simulink model "two_sub_model"  (Simulink 8.4)
settings: Solver=FixedStepDiscrete  StartTime=0.0  StopTime="                                                                                 300"  FixedStep=1/256  RelTol=1e-3
undefined symbols (not defined in the file): currentCFG_one_sub_model_UB, UB
libraries: gRTanalyze x6, gUSBamplib x2, Tools x1
settings Model: Creator=2110973l  LastModifiedBy=2110973l
settings DataIOCC: SignalLoggingSaveFormat=Dataset
settings OptimizationCC: ExpressionDepthLimit=128
settings DebuggingCC: UnderspecifiedInitializationDetection=Simplified  MergeDetectMultiDrivingBlocksExec=error  FcnCallInpInsideContextMsg=EnableAllAsError  StateNameClashWarn=none
settings GRTTargetCC: CombineOutputUpdateFcns=on  GRTInterface=off

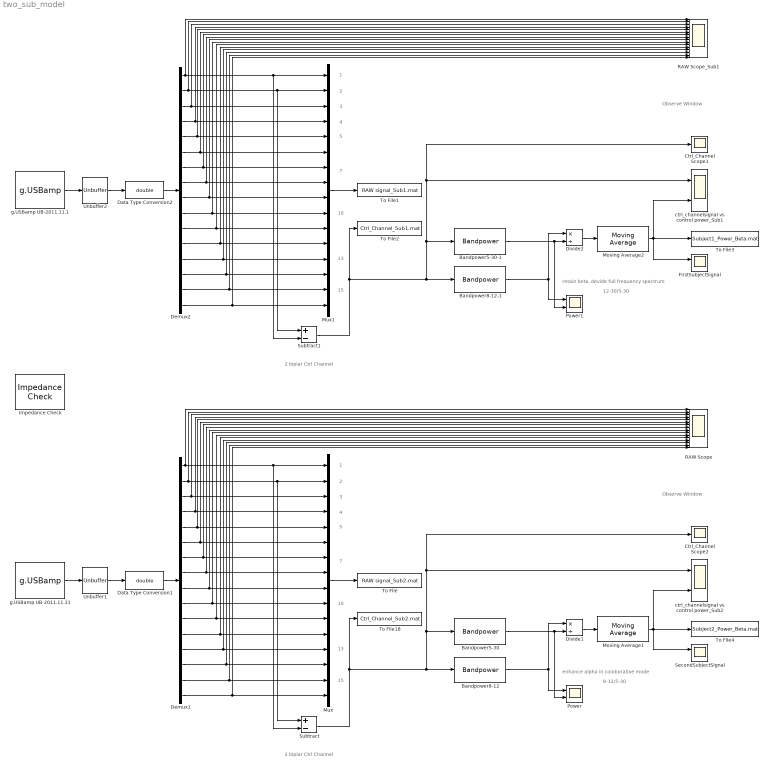
== system two_sub_model ==
  note: 13
  note: 15
  note: 4
  note: 3
  note: 7
  note: 10
  note: 5
  note: 2
  note: 1
  note: Observe Window
  note: 2 biplar Ctrl Channel
  note: enhance alpha in coloborative mode
  note: 8-12/5-30
  note: 13
  note: 15
  note: 4
  note: 3
  note: 7
  note: 10
  note: 5
  note: 2
  note: 1
  note: Observe Window
  note: 2 biplar Ctrl Channel
  note: retain beta, devide full frequency spectrum
  note: 12-30/5-30
  Bandpower5-30 : gRTanalyze/Bandpower  Order=5  LowerFreq=5  UpperFreq=30  WindowLength=128
  Bandpower5-30-1 : gRTanalyze/Bandpower  Order=5  LowerFreq=5  UpperFreq=30  WindowLength=128
  Bandpower8-12 : gRTanalyze/Bandpower  Order=5  LowerFreq=8  UpperFreq=12  WindowLength=128
  Bandpower8-12-1 : gRTanalyze/Bandpower  Order=5  LowerFreq=8  UpperFreq=12  WindowLength=128
  Ctrl_Channel Scope1 : Scope
      settings: YMin=-100  YMax=100  SaveName=ScopeData2
  Ctrl_Channel Scope2 : Scope
      settings: YMin=-100  YMax=100
  Data Type Conversion1 : DataTypeConversion  OutDataTypeStr=double
  Data Type Conversion2 : DataTypeConversion  OutDataTypeStr=double
  Demux1 : Demux  Outputs=16
  Demux2 : Demux  Outputs=16
  Divide1 : Product  Inputs=*/
  Divide2 : Product  Inputs=*/
  FirstSubjectSignal : Scope  NumInputPorts=2
      settings: YMin=1.014~-1  YMax=1.032~1  SaveName=ScopeData8
  Impedance Check : Tools/Impedance Check  SystemSampleTime=-1
  Moving Average1 : gRTanalyze/Moving Average  windowSize=256
  Moving Average2 : gRTanalyze/Moving Average  windowSize=256
  Mux : Mux  Inputs=16
  Mux1 : Mux  Inputs=16
  Power : Scope  NumInputPorts=2
      settings: YMin=0~0  YMax=1200~1200  SaveName=ScopeData5
  Power1 : Scope  NumInputPorts=2
      settings: YMin=0~0  YMax=1200~1200  SaveName=ScopeData4
  RAW Scope : Scope  NumInputPorts=16
      settings: YMin=-50~-50~-50~-50~-50~-50~-50~-50~-50~-50~-50~-50~-100~-50~-100~-100  YMax=50~50~50~50~50~50~50~50~50~50~50~50~100~50~100~100
  RAW Scope_Sub1 : Scope  NumInputPorts=16
      settings: YMin=-50~-50~-50~-50~-50~-50~-50~-50~-50~-50~-50~-50~-100~-50~-100~-100  YMax=50~50~50~50~50~50~50~50~50~50~50~50~100~50~100~100  SaveName=ScopeData6
  SecondSubjectSignal : Scope  NumInputPorts=2
      settings: YMin=1.014~-1  YMax=1.032~1  SaveName=ScopeData3
  Subtract : Sum  Inputs=+-
  Subtract1 : Sum  Inputs=+-
  To File : ToFile  Filename=RAW signal_Sub2.mat  MatrixName=AllChannel
  To File1 : ToFile  Filename=RAW signal_Sub1.mat  MatrixName=AllChannel
  To File18 : ToFile  Filename=Ctrl_Channel_Sub2.mat  MatrixName=Ctrl_Channel
  To File2 : ToFile  Filename=Ctrl_Channel_Sub1.mat  MatrixName=Ctrl_Channel
  To File3 : ToFile  Filename=Subject1_Power_Beta.mat  MatrixName=Subject1_Power_Beta
  To File4 : ToFile  Filename=Subject2_Power_Beta.mat  MatrixName=Subject2_Power_Beta
  Unbuffer1 : Unbuffer  SampleBasedProcessing=Same as frame based
  Unbuffer2 : Unbuffer  SampleBasedProcessing=Same as frame based
  ctrl_channelsignal vs control power_Sub1 : Scope  NumInputPorts=2
      settings: YMin=-100~0  YMax=100~20  SaveName=ScopeData9
  ctrl_channelsignal vs control power_Sub2 : Scope  NumInputPorts=2
      settings: YMin=-100~0  YMax=100~20  SaveName=ScopeData7
  g.USBamp UB-2011.11.1 : gUSBamplib/g.USBamp  cfg=currentCFG_one_sub_model_UB-2011.11.31.cfg  snr=UB-2011.11.31
  g.USBamp UB-2011.11.31 : gUSBamplib/g.USBamp  cfg=currentCFG_one_sub_model_UB-2011.11.31.cfg  snr=UB-2011.11.31
  wires:
  Bandpower8-12/1 -> Divide1/1, Power/1
  Bandpower5-30/1 -> Divide1/2, Power/2
  Moving Average1/1 -> To File4/1, ctrl_channelsignal vs control power_Sub2/2, SecondSubjectSignal/1
  Divide1/1 -> Moving Average1/1
  g.USBamp UB-2011.11.31/1 -> Unbuffer1/1
  Unbuffer1/1 -> Data Type Conversion1/1
  Data Type Conversion1/1 -> Demux1/1
  Demux1/11 -> RAW Scope/11, Mux/11
  Demux1/13 -> RAW Scope/13, Mux/13
  Demux1/15 -> RAW Scope/15, Mux/15
  Demux1/1 -> Subtract/2, Mux/1, RAW Scope/1
  Demux1/7 -> RAW Scope/7, Mux/7
  Demux1/9 -> RAW Scope/9, Mux/9
  Subtract/1 -> Bandpower8-12/1, Bandpower5-30/1, Ctrl_Channel Scope2/1, ctrl_channelsignal vs control power_Sub2/1, To File18/1
  Demux1/2 -> Subtract/1, Mux/2, RAW Scope/2
  Demux1/4 -> Mux/4, RAW Scope/4
  Demux1/6 -> RAW Scope/6, Mux/6
  Demux1/8 -> RAW Scope/8, Mux/8
  Demux1/12 -> RAW Scope/12, Mux/12
  Demux1/14 -> RAW Scope/14, Mux/14
  Demux1/16 -> RAW Scope/16, Mux/16
  Demux1/5 -> RAW Scope/5, Mux/5
  Demux1/3 -> Mux/3, RAW Scope/3
  Demux1/10 -> RAW Scope/10, Mux/10
  Mux/1 -> To File/1
  Bandpower8-12-1/1 -> Divide2/1, Power1/1
  Bandpower5-30-1/1 -> Divide2/2, Power1/2
  Moving Average2/1 -> To File3/1, ctrl_channelsignal vs control power_Sub1/2, FirstSubjectSignal/1
  Divide2/1 -> Moving Average2/1
  g.USBamp UB-2011.11.1/1 -> Unbuffer2/1
  Unbuffer2/1 -> Data Type Conversion2/1
  Data Type Conversion2/1 -> Demux2/1
  Demux2/11 -> RAW Scope_Sub1/11, Mux1/11
  Demux2/13 -> RAW Scope_Sub1/13, Mux1/13
  Demux2/15 -> RAW Scope_Sub1/15, Mux1/15
  Demux2/1 -> Subtract1/2, Mux1/1, RAW Scope_Sub1/1
  Demux2/7 -> RAW Scope_Sub1/7, Mux1/7
  Demux2/9 -> RAW Scope_Sub1/9, Mux1/9
  Subtract1/1 -> Bandpower8-12-1/1, Bandpower5-30-1/1, Ctrl_Channel Scope1/1, ctrl_channelsignal vs control power_Sub1/1, To File2/1
  Demux2/2 -> Subtract1/1, Mux1/2, RAW Scope_Sub1/2
  Demux2/4 -> Mux1/4, RAW Scope_Sub1/4
  Demux2/6 -> RAW Scope_Sub1/6, Mux1/6
  Demux2/8 -> RAW Scope_Sub1/8, Mux1/8
  Demux2/12 -> RAW Scope_Sub1/12, Mux1/12
  Demux2/14 -> RAW Scope_Sub1/14, Mux1/14
  Demux2/16 -> RAW Scope_Sub1/16, Mux1/16
  Demux2/5 -> RAW Scope_Sub1/5, Mux1/5
  Demux2/3 -> Mux1/3, RAW Scope_Sub1/3
  Demux2/10 -> RAW Scope_Sub1/10, Mux1/10
  Mux1/1 -> To File1/1
